simulink model "Simscape_Benchmark_SIM1"  (R2021a)
settings: Solver=ode45  StartTime=0.0  StopTime=PHASE.Ttotal  FixedStep=Benchmark.Sim.Tint  RelTol=1e-5  AbsTol=1e-6
undefined symbols (not defined in the file): Actuators, Analysis, antisym, Benchmark, Bus, Disturbance, FSM, IntialCond, ISOL, K_Coarse_disc_t, Kslew_opt_disc_zoh, Model, MPS, PAYLOAD, PHASE, PMA, RWIsol, RWS, SA, Sensors, Slew, slosh, thr, X, Y, Z
libraries: sm_lib x215, nesl_utility x148, simulink x65, cstblocks x36, sharedtransform x4, vrlib x3, RCTblocks x1
(part 4 of 9)

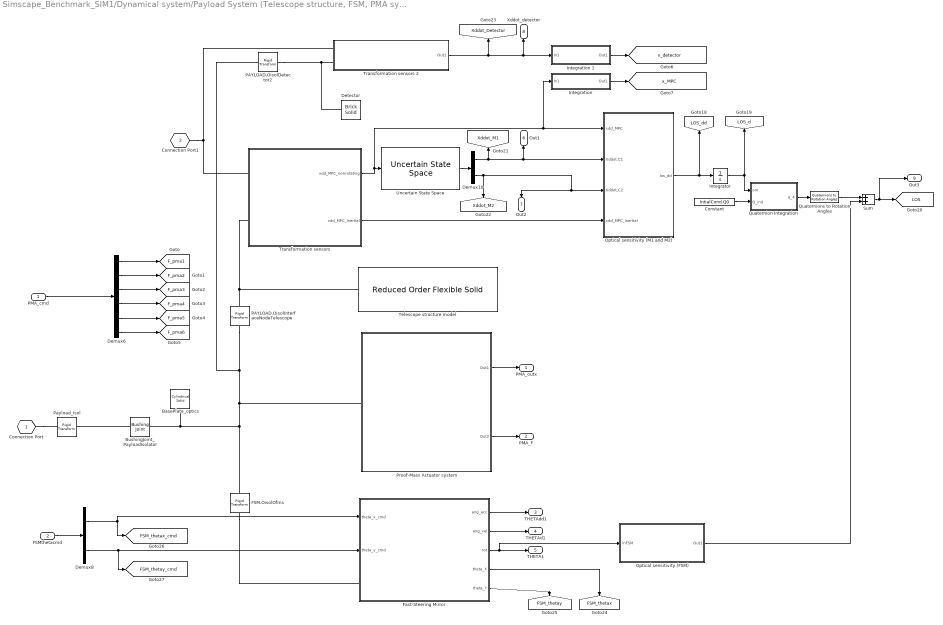
== system Simscape_Benchmark_SIM1/Dynamical system/Payload System (Telescope structure, FSM, PMA system, Isolator) ==
  PMA_cmd : Inport
  FSMthetacmd : Inport  Port=2
  BasePlate_optics : sm_lib/Body Elements/Cylindrical Solid  GraphicAmbientColor=[0.15 0.15 0.15 1.0]  BasedOnType=Density  CenterOfMass=[0;0;0]  CenterOfMassUnits=m  GraphicDiffuseColor=[0.0 0.2 0.6]  CylinderLength=ISOL.SIM.length  CylinderLengthUnits=m  CylinderRadius=ISOL.SIM.r_visualization  CylinderRadiusUnits=m  Density=1000  DensityUnits=kg/m^3  DoExposeReferenceFrame=off  GraphicEmissiveColor=[0.0 0.0 0.0 1.0]  ExportEntireGeometry=off  SerializedFrames=<Frames><Frame><Id>Frame1</Id><Value><Name>F1</Name><Origin><Source>GeometricFeature</Source><FeatureName>bottom surface</FeatureName></Origin><PrimaryAxis><DefinedDirection>+Z</DefinedDirection><Source>ReferenceFrame</Source><SourceDirection>+Z</SourceDirection><FeatureName></FeatureName></PrimaryAxis><SecondaryAxis><DefinedDirection>+X</DefinedDirection><Source>ReferenceFrame</Source><SourceDirection>+X</SourceDirection><FeatureName></FeatureName></SecondaryAxis></Value></Frame></Frames>  MarkerShape=Sphere  MarkerSize=10  GraphicType=FromGeometry  InertiaType=Custom  Mass=ISOL.m_simscape  MassUnits=kg  MomentsOfInertia=diag(ISOL.IatG_simscape)  MomentsOfInertiaUnits=kg*m^2  GraphicOpacity=0.4  ProductsOfInertia=[ISOL.IatG_simscape(2,3),ISOL.IatG_simscape(1,3),ISOL.IatG_simscape(1,2)]'  ProductsOfInertiaUnits=kg*m^2  GraphicShininess=75  GraphicSpecularColor=[0.5 0.5 0.5 1.0]  GraphicVisPropType=SimpleVisualProperties
  BushingJoint_PayloadIsolator : sm_lib/Joints/Bushing Joint  JointMode=Normal  SenseConstraintForce=off  SenseConstraintForceX=off  SenseConstraintForceY=off  SenseConstraintForceZ=off  SenseConstraintTorque=off  SenseConstraintTorqueX=off  SenseConstraintTorqueY=off  SenseConstraintTorqueZ=off  SenseTotalForce=off  SenseTotalForceX=off  SenseTotalForceY=off  SenseTotalForceZ=off  SenseTotalTorque=off  SenseTotalTorqueX=off  SenseTotalTorqueY=off  SenseTotalTorqueZ=off  CompositeWrenchDir=FollowerOnBase  CompositeWrenchFrame=BaseFrame  PxEquilibriumPosition=0  PxEquilibriumPositionUnits=m  PxSpringStiffness=ISOL.K(1,1)  PxSpringStiffnessUnits=N/m  PxDampingCoefficient=ISOL.D(1,1)  PxDampingCoefficientUnits=N/(m/s)  PxTorqueActuationMode=NoTorque  PxMotionActuationMode=ComputedMotion  PxSensePosition=off  PxSenseVelocity=off  PxSenseAcceleration=off  PxSenseTorqueForce=off  PxSenseLowerLimitTorqueForce=off  PxSenseUpperLimitTorqueForce=off  PxLowerLimitSpecify=off  PxLowerLimitBound=-1  PxLowerLimitBoundUnits=m  PxLowerLimitStiffness=1e6  PxLowerLimitStiffnessUnits=N/m  PxLowerLimitDamping=1e3  PxLowerLimitDampingUnits=N/(m/s)  PxLowerLimitTransitionRegionWidth=1e-4  PxLowerLimitTransitionRegionWidthUnits=m  PxUpperLimitSpecify=off  PxUpperLimitBound=1  PxUpperLimitBoundUnits=m  PxUpperLimitStiffness=1e6  PxUpperLimitStiffnessUnits=N/m  PxUpperLimitDamping=1e3  PxUpperLimitDampingUnits=N/(m/s)  PxUpperLimitTransitionRegionWidth=1e-4  PxUpperLimitTransitionRegionWidthUnits=m  PxPositionTargetSpecify=off  PxPositionTargetPriority=High  PxPositionTargetValue=0  PxPositionTargetValueUnits=m  PxVelocityTargetSpecify=off  PxVelocityTargetPriority=High  PxVelocityTargetValue=0  PxVelocityTargetValueUnits=m/s  PyEquilibriumPosition=0  PyEquilibriumPositionUnits=m  PySpringStiffness=ISOL.K(2,2)  PySpringStiffnessUnits=N/m  PyDampingCoefficient=ISOL.D(2,2)  PyDampingCoefficientUnits=N/(m/s)  PyTorqueActuationMode=NoTorque  PyMotionActuationMode=ComputedMotion  PySensePosition=off  PySenseVelocity=off  PySenseAcceleration=off  PySenseTorqueForce=off  PySenseLowerLimitTorqueForce=off  PySenseUpperLimitTorqueForce=off  PyLowerLimitSpecify=on  PyLowerLimitBound=-1  PyLowerLimitBoundUnits=m  PyLowerLimitStiffness=1e6  PyLowerLimitStiffnessUnits=N/m  PyLowerLimitDamping=1e3  PyLowerLimitDampingUnits=N/(m/s)  PyLowerLimitTransitionRegionWidth=1e-4  PyLowerLimitTransitionRegionWidthUnits=m  PyUpperLimitSpecify=off  PyUpperLimitBound=1  PyUpperLimitBoundUnits=m  PyUpperLimitStiffness=1e6  PyUpperLimitStiffnessUnits=N/m  PyUpperLimitDamping=1e3  PyUpperLimitDampingUnits=N/(m/s)  PyUpperLimitTransitionRegionWidth=1e-4  PyUpperLimitTransitionRegionWidthUnits=m  PyPositionTargetSpecify=off  PyPositionTargetPriority=High  PyPositionTargetValue=0  PyPositionTargetValueUnits=m  PyVelocityTargetSpecify=off  PyVelocityTargetPriority=High  PyVelocityTargetValue=0  PyVelocityTargetValueUnits=m/s  PzEquilibriumPosition=0  PzEquilibriumPositionUnits=m  PzSpringStiffness=ISOL.K(3,3)  PzSpringStiffnessUnits=N/m  PzDampingCoefficient=ISOL.D(3,3)  PzDampingCoefficientUnits=N/(m/s)  PzTorqueActuationMode=NoTorque  PzMotionActuationMode=ComputedMotion  PzSensePosition=off  PzSenseVelocity=off  PzSenseAcceleration=off  PzSenseTorqueForce=off  PzSenseLowerLimitTorqueForce=off  PzSenseUpperLimitTorqueForce=off  PzLowerLimitSpecify=off  PzLowerLimitBound=-1  PzLowerLimitBoundUnits=m  PzLowerLimitStiffness=1e6  PzLowerLimitStiffnessUnits=N/m  PzLowerLimitDamping=1e3  PzLowerLimitDampingUnits=N/(m/s)  PzLowerLimitTransitionRegionWidth=1e-4  PzLowerLimitTransitionRegionWidthUnits=m  PzUpperLimitSpecify=off  PzUpperLimitBound=1  PzUpperLimitBoundUnits=m  PzUpperLimitStiffness=1e6  PzUpperLimitStiffnessUnits=N/m  PzUpperLimitDamping=1e3  PzUpperLimitDampingUnits=N/(m/s)  PzUpperLimitTransitionRegionWidth=1e-4  PzUpperLimitTransitionRegionWidthUnits=m  PzPositionTargetSpecify=off  PzPositionTargetPriority=High  PzPositionTargetValue=0  PzPositionTargetValueUnits=m  PzVelocityTargetSpecify=off  PzVelocityTargetPriority=High  PzVelocityTargetValue=0  PzVelocityTargetValueUnits=m/s  RxEquilibriumPosition=0  RxEquilibriumPositionUnits=deg  RxSpringStiffness=ISOL.K(4,4)  RxSpringStiffnessUnits=N*m/rad  RxDampingCoefficient=ISOL.D(4,4)  RxDampingCoefficientUnits=N*m/(rad/s)  RxTorqueActuationMode=NoTorque  RxMotionActuationMode=ComputedMotion  RxSensePosition=off  RxSenseVelocity=off  RxSenseAcceleration=off  RxSenseTorqueForce=off  RxSenseLowerLimitTorqueForce=off  RxSenseUpperLimitTorqueForce=off  RxLowerLimitSpecify=off  RxLowerLimitBound=-90  RxLowerLimitBoundUnits=deg  RxLowerLimitStiffness=1e4  RxLowerLimitStiffnessUnits=N*m/deg  RxLowerLimitDamping=10  RxLowerLimitDampingUnits=N*m/(deg/s)  RxLowerLimitTransitionRegionWidth=0.1  RxLowerLimitTransitionRegionWidthUnits=deg  RxUpperLimitSpecify=off  RxUpperLimitBound=90  RxUpperLimitBoundUnits=deg  RxUpperLimitStiffness=1e4  RxUpperLimitStiffnessUnits=N*m/deg  RxUpperLimitDamping=10  RxUpperLimitDampingUnits=N*m/(deg/s)  RxUpperLimitTransitionRegionWidth=0.1  RxUpperLimitTransitionRegionWidthUnits=deg  RxPositionTargetSpecify=off  RxPositionTargetPriority=High  RxPositionTargetValue=0  RxPositionTargetValueUnits=deg  RxVelocityTargetSpecify=off  RxVelocityTargetPriority=High  RxVelocityTargetValue=0  RxVelocityTargetValueUnits=deg/s  RyEquilibriumPosition=0  RyEquilibriumPositionUnits=deg  RySpringStiffness=ISOL.K(5,5)  RySpringStiffnessUnits=N*m/rad  RyDampingCoefficient=ISOL.D(5,5)  RyDampingCoefficientUnits=N*m/(rad/s)  RyTorqueActuationMode=NoTorque  RyMotionActuationMode=ComputedMotion  RySensePosition=off  RySenseVelocity=off  RySenseAcceleration=off  RySenseTorqueForce=off  RySenseLowerLimitTorqueForce=off  RySenseUpperLimitTorqueForce=off  RyLowerLimitSpecify=off  RyLowerLimitBound=-90  RyLowerLimitBoundUnits=deg  RyLowerLimitStiffness=1e4  RyLowerLimitStiffnessUnits=N*m/deg  RyLowerLimitDamping=10  RyLowerLimitDampingUnits=N*m/(deg/s)  RyLowerLimitTransitionRegionWidth=0.1  RyLowerLimitTransitionRegionWidthUnits=deg  RyUpperLimitSpecify=off  RyUpperLimitBound=90  RyUpperLimitBoundUnits=deg  RyUpperLimitStiffness=1e4  RyUpperLimitStiffnessUnits=N*m/deg  RyUpperLimitDamping=10  RyUpperLimitDampingUnits=N*m/(deg/s)  RyUpperLimitTransitionRegionWidth=0.1  RyUpperLimitTransitionRegionWidthUnits=deg  RyPositionTargetSpecify=off  RyPositionTargetPriority=High  RyPositionTargetValue=0  RyPositionTargetValueUnits=deg  RyVelocityTargetSpecify=off  RyVelocityTargetPriority=High  RyVelocityTargetValue=0  RyVelocityTargetValueUnits=deg/s  RzEquilibriumPosition=0  RzEquilibriumPositionUnits=deg  RzSpringStiffness=ISOL.K(6,6)  RzSpringStiffnessUnits=N*m/rad  RzDampingCoefficient=ISOL.D(6,6)  RzDampingCoefficientUnits=N*m/(rad/s)  RzTorqueActuationMode=NoTorque  RzMotionActuationMode=ComputedMotion  RzSensePosition=off  RzSenseVelocity=off  RzSenseAcceleration=off  RzSenseTorqueForce=off  RzSenseLowerLimitTorqueForce=off  RzSenseUpperLimitTorqueForce=off  RzLowerLimitSpecify=off  RzLowerLimitBound=-90  RzLowerLimitBoundUnits=deg  RzLowerLimitStiffness=1e4  RzLowerLimitStiffnessUnits=N*m/deg  RzLowerLimitDamping=10  RzLowerLimitDampingUnits=N*m/(deg/s)  RzLowerLimitTransitionRegionWidth=0.1  RzLowerLimitTransitionRegionWidthUnits=deg  RzUpperLimitSpecify=off  RzUpperLimitBound=90  RzUpperLimitBoundUnits=deg  RzUpperLimitStiffness=1e4  RzUpperLimitStiffnessUnits=N*m/deg  RzUpperLimitDamping=10  RzUpperLimitDampingUnits=N*m/(deg/s)  RzUpperLimitTransitionRegionWidth=0.1  RzUpperLimitTransitionRegionWidthUnits=deg  RzPositionTargetSpecify=off  RzPositionTargetPriority=High  RzPositionTargetValue=0  RzPositionTargetValueUnits=deg  RzVelocityTargetSpecify=off  RzVelocityTargetPriority=High  RzVelocityTargetValue=0  RzVelocityTargetValueUnits=deg/s
  Constant : Constant  Value=IntialCond.Q0
  Demux10 : Demux  Outputs=[6,6]
  Demux6 : Demux  Outputs=6
  Demux8 : Demux  Outputs=2
  Detector : sm_lib/Body Elements/Brick Solid  GraphicAmbientColor=[0.15 0.15 0.15 1.0]  BasedOnType=Density  BrickDimensions=[0.05 0.05 0.002]  BrickDimensionUnits=m  CenterOfMass=[0 0 0]  CenterOfMassUnits=m  GraphicDiffuseColor=[1.0 1.0 0.0]  Density=0  DensityUnits=kg/m^3  DoExposeReferenceFrame=on  GraphicEmissiveColor=[0.0 0.0 0.0 1.0]  ExportEntireGeometry=off  SerializedFrames=<Frames/>  MarkerShape=Sphere  MarkerSize=10  GraphicType=FromGeometry  InertiaType=CalculateFromGeometry  Mass=1  MassUnits=kg  MomentsOfInertia=[1 1 1]  MomentsOfInertiaUnits=kg*m^2  GraphicOpacity=1.0  ProductsOfInertia=[0 0 0]  ProductsOfInertiaUnits=kg*m^2  GraphicShininess=75  GraphicSpecularColor=[0.5 0.5 0.5 1.0]  GraphicVisPropType=SimpleVisualProperties
  FSM.OisolOfms : sm_lib/Frames and Transforms/Rigid Transform  TranslationMethod=Cartesian  TranslationStandardOffset=0  TranslationLengthUnit=m  TranslationStandardAxis=+Z  TranslationCartesianOffset=FSM.OisolOfms  TranslationROffset=0  TranslationROffsetUnits=m  TranslationZOffset=0  TranslationZOffsetUnits=m  TranslationThetaOffset=0  TranslationThetaOffsetUnits=deg  RotationMethod=RotationMatrix  RotationAngleUnits=deg  RotationStandardAxis=+Z  RotationAngle=0.0  RotationArbitraryAxis=[0 0 1]  FollAlignAxisA=+X  BaseAlignAxisA=+Y  FollAlignAxisB=+Y  BaseAlignAxisB=+Z  RotationSequenceAxes=FollowerAxes  RotationSequence=XYX  RotationSequenceAngles=[0 0 0]  RotationSequenceAnglesUnits=deg  RotationMatrix=FSM.DCM
  Fast-Steering Mirror : Subsystem
  Integration : Subsystem
  Integration 1 : Subsystem
  Integrator : Integrator
  Optical sensitivity (FSM) : Subsystem
  Optical sensitivity (M1 and M2) : Subsystem
  PAYLOAD.OisolDetector2 : sm_lib/Frames and Transforms/Rigid Transform  TranslationMethod=Cartesian  TranslationStandardOffset=0  TranslationLengthUnit=m  TranslationStandardAxis=+Z  TranslationCartesianOffset=PAYLOAD.Detector.OisolDetector  TranslationROffset=0  TranslationROffsetUnits=m  TranslationZOffset=0  TranslationZOffsetUnits=m  TranslationThetaOffset=0  TranslationThetaOffsetUnits=deg  RotationMethod=RotationMatrix  RotationAngleUnits=deg  RotationStandardAxis=+Z  RotationAngle=0.0  RotationArbitraryAxis=[0 0 1]  FollAlignAxisA=+X  BaseAlignAxisA=+Y  FollAlignAxisB=+Y  BaseAlignAxisB=+Z  RotationSequenceAxes=FollowerAxes  RotationSequence=XYX  RotationSequenceAngles=[0 0 0]  RotationSequenceAnglesUnits=deg  RotationMatrix=PAYLOAD.Detector.DCM
  PAYLOAD.OisolInterfaceNodeTelescope : sm_lib/Frames and Transforms/Rigid Transform  TranslationMethod=Cartesian  TranslationStandardOffset=0  TranslationLengthUnit=m  TranslationStandardAxis=+Z  TranslationCartesianOffset=PAYLOAD.OisolInterfaceNodeTelescope  TranslationROffset=0  TranslationROffsetUnits=m  TranslationZOffset=0  TranslationZOffsetUnits=m  TranslationThetaOffset=0  TranslationThetaOffsetUnits=deg  RotationMethod=None  RotationAngleUnits=deg  RotationStandardAxis=+Z  RotationAngle=0.0  RotationArbitraryAxis=[0 0 1]  FollAlignAxisA=+X  BaseAlignAxisA=+Y  FollAlignAxisB=+Y  BaseAlignAxisB=+Z  RotationSequenceAxes=FollowerAxes  RotationSequence=XYX  RotationSequenceAngles=[0 0 0]  RotationSequenceAnglesUnits=deg  RotationMatrix=[1 0 0; 0 1 0; 0 0 1]
  Payload_Isol : sm_lib/Frames and Transforms/Rigid Transform  TranslationMethod=Cartesian  TranslationStandardOffset=0  TranslationLengthUnit=m  TranslationStandardAxis=+Z  TranslationCartesianOffset=ISOL.ObP  TranslationROffset=0  TranslationROffsetUnits=m  TranslationZOffset=0  TranslationZOffsetUnits=m  TranslationThetaOffset=0  TranslationThetaOffsetUnits=deg  RotationMethod=None  RotationAngleUnits=deg  RotationStandardAxis=+Z  RotationAngle=0.0  RotationArbitraryAxis=[0 0 1]  FollAlignAxisA=+X  BaseAlignAxisA=+Y  FollAlignAxisB=+Y  BaseAlignAxisB=+Z  RotationSequenceAxes=FollowerAxes  RotationSequence=XYX  RotationSequenceAngles=[0 0 0]  RotationSequenceAnglesUnits=deg  RotationMatrix=[1 0 0; 0 1 0; 0 0 1]
  Proof-Mass Actuator system : Subsystem
  Quaternion Integration : Subsystem
  Quaternions to Rotation Angles : sharedtransform/Quaternions to Rotation Angles  rotationOrder=XYZ  aMode=aMode
      settings: SourceProductBaseCode=AE,PW,DR,MT,UV,VE
  Sum : Sum
  Telescope structure model : sm_lib/Body Elements/Flexible Bodies/Reduced Order Flexible Solid  GraphicAmbientColor=[0.15 0.15 0.15 1.0]  GraphicDiffuseColor=[0.0 0.2 0.6]  DampingType=DampingMatrix  GraphicEmissiveColor=[0.0 0.0 0.0 1.0]  GeomFileName=file_telescope.stl  GraphicType=PartitionedGeometry  MassMatrix=PAYLOAD.Mrofs_telescopeSIMULATOR  NumberOfInterfaceFrames=1  GraphicOpacity=1  InterfaceFrameOrigins=PAYLOAD.coord_telescopeSIMULATOR  GraphicShininess=0  GraphicSpecularColor=[0.5 0.5 0.5 1.0]  StiffnessMatrix=PAYLOAD.Krofs_telescopeSIMULATOR  GeomUnitType=FromUnitSystem  VisRecursionLimit=3  GraphicVisPropType=SimpleVisualProperties  LengthUnit=m  MassUnit=kg  TimeUnit=s  UnitSystemType=SI  ProportionalDampingAlpha=0  ProportionalDampingBeta=0.001  UniformModalDampingRatio=0.005  DampingMatrix=PAYLOAD.Drofs_telescopeSIMULATOR
      settings: SourceProductBaseCode=MS
  Transformation sensors : Subsystem
  Transformation sensors 2 : Subsystem
  Uncertain State Space : RCTblocks/Uncertain State Space  Tag=USS  USystem=TF_telescope  UValue=PAYLOAD.Struct  X0=[]  uX0=[]
      settings: SourceProductBaseCode=RC
  Connection Port : PMIOPort  Tag=PMCPort  Side=Left
  Connection Port1 : PMIOPort  Tag=PMCPort  Port=2  Side=Left
  PMA_outx : Outport
  PMA_F : Outport  Port=2
  THETAdd1 : Outport  Port=3
  THETAd1 : Outport  Port=4
  THETA1 : Outport  Port=5
  Out1 : Outport  Port=6
  Out2 : Outport  Port=7
  Xddot_detector : Outport  Port=8
  Out3 : Outport  Port=9
  tag scope: FSM_thetax=global, FSM_thetax_cmd=global, FSM_thetay=global, FSM_thetay_cmd=global, F_pma1=global, F_pma2=global, F_pma3=global, F_pma4=global, F_pma5=global, F_pma6=global, LOS=global, LOS_d=global, LOS_dd=global, Xddot_Detector=global, Xddot_M1=global, Xddot_M2=global, x_MPC=global, x_detector=global
  wires:
  Demux6/2 -> [F_pma2]
  PMA_cmd/1 -> Demux6/1
  Demux6/1 -> [F_pma1]
  Demux6/6 -> [F_pma6]
  Demux6/5 -> [F_pma5]
  Demux6/3 -> [F_pma3]
  Demux6/4 -> [F_pma4]
  Demux8/2 -> [FSM_thetay_cmd], Fast-Steering Mirror/2(theta_y_cmd)
  Demux10/1 -> Optical sensitivity (M1 and M2)/2(Xddot,C1), Out1/1, [Xddot_M1]
  Optical sensitivity (M1 and M2)/1(los_dd) -> Integrator/1, [LOS_dd]
  Uncertain State Space/1 -> Demux10/1
  Demux8/1 -> [FSM_thetax_cmd], Fast-Steering Mirror/1(theta_x_cmd)
  Sum/1 -> Out3/1, [LOS]
  FSMthetacmd/1 -> Demux8/1
  Proof-Mass Actuator system/1(Out1) -> PMA_outx/1
  Proof-Mass Actuator system/2(Out2) -> PMA_F/1
  Fast-Steering Mirror/3(rot) -> Optical sensitivity (FSM)/1(inFSM), THETA1/1
  Fast-Steering Mirror/1(ang_acc) -> THETAdd1/1
  Fast-Steering Mirror/2(ang_vel) -> THETAd1/1
  Fast-Steering Mirror/4(theta_X) -> [FSM_thetax]
  Fast-Steering Mirror/5(theta_Y) -> [FSM_thetay]
  Demux10/2 -> Out2/1, Optical sensitivity (M1 and M2)/3(Xddot,C2), [Xddot_M2]
  Constant/1 -> Quaternion Integration/2(Q_init)
  Integrator/1 -> Quaternion Integration/1(om), [LOS_d]
  Quaternion Integration/1(q_4) -> Quaternions to Rotation Angles/1
  Optical sensitivity (FSM)/1(Out1) -> Sum/2
  Quaternions to Rotation Angles/1 -> Sum/1
  Integration/1(Out1) -> [x_MPC]
  Integration 1/1(Out1) -> [x_detector]
  Transformation sensors/1(xdd_MPC_nonrotating) -> Optical sensitivity (M1 and M2)/1(xdd_MPC), Integration/1(In1), Uncertain State Space/1
  Transformation sensors/2(xdd_MPC_Inertial) -> Optical sensitivity (M1 and M2)/4(xdd_MPC_Inertial)
  Transformation sensors 2/1(Out1) -> [Xddot_Detector], Xddot_detector/1, Integration 1/1(In1)
  connections:
  Connection Port/RConn1 -- Payload_Isol/LConn1
  FSM.OisolOfms/LConn1 -- PAYLOAD.OisolInterfaceNodeTelescope/LConn1 -- PAYLOAD.OisolDetector2/LConn1 -- Proof-Mass Actuator system/LConn1 -- BushingJoint_PayloadIsolator/RConn1 -- BasePlate_optics/LConn1
  BushingJoint_PayloadIsolator/LConn1 -- Payload_Isol/RConn1
  PAYLOAD.OisolInterfaceNodeTelescope/RConn1 -- Telescope structure model/LConn1 -- Transformation sensors/LConn2
  FSM.OisolOfms/RConn1 -- Fast-Steering Mirror/LConn1
  PAYLOAD.OisolDetector2/RConn1 -- Transformation sensors 2/LConn2 -- Detector/RConn1
  Connection Port1/RConn1 -- Transformation sensors/LConn1 -- Transformation sensors 2/LConn1

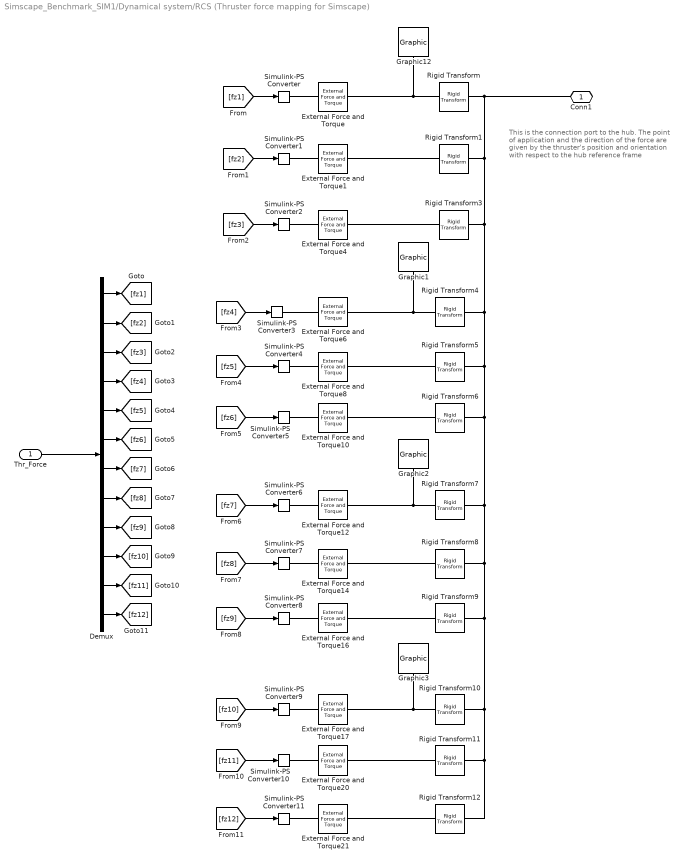
== system Simscape_Benchmark_SIM1/Dynamical system/RCS (Thruster force mapping for Simscape) ==
  note: This is the connection port to the hub. The point of application
      | and the direction of the force are given by the thruster's position
      | and orientation with respect to the hub reference frame
  Thr_Force : Inport
  Demux : Demux  Outputs=12
  External Force and Torque{,1,4,6,8,10,12,14,16..17,20..21} (12 alike) : sm_lib/Forces and Torques/External Force and Torque  ForceResolutionFrame=AttachedFrame  EnableForceX=off  EnableForceY=off  EnableForceZ=on  EnableForce=off  TorqueResolutionFrame=AttachedFrame  EnableTorqueX=off  EnableTorqueY=off  EnableTorqueZ=off  EnableTorque=off
  Graphic{1..3,12} (4 alike) : sm_lib/Body Elements/Graphic  GraphicType=Marker  MarkerShape=Frame  MarkerSize=15  GraphicVisPropType=SimpleVisualProperties  GraphicDiffuseColor=[0.0 0.0 0.8]  GraphicSpecularColor=[0.5 0.5 0.5 1.0]  GraphicAmbientColor=[0.15 0.15 0.15 1.0]  GraphicEmissiveColor=[0.0 0.0 0.0 1.0]  GraphicShininess=75  GraphicOpacity=1.0
  Rigid Transform : sm_lib/Frames and Transforms/Rigid Transform  TranslationMethod=Cartesian  TranslationStandardOffset=0  TranslationLengthUnit=m  TranslationStandardAxis=+Z  TranslationCartesianOffset=thr.sc_thrust_pos(:,1)  TranslationROffset=0  TranslationROffsetUnits=m  TranslationZOffset=0  TranslationZOffsetUnits=m  TranslationThetaOffset=0  TranslationThetaOffsetUnits=deg  RotationMethod=RotationMatrix  RotationAngleUnits=deg  RotationStandardAxis=+Z  RotationAngle=0.0  RotationArbitraryAxis=[0 0 1]  FollAlignAxisA=+X  BaseAlignAxisA=+Y  FollAlignAxisB=+Y  BaseAlignAxisB=+Z  RotationSequenceAxes=FollowerAxes  RotationSequence=XYX  RotationSequenceAngles=[0 0 0]  RotationSequenceAnglesUnits=deg  RotationMatrix=thr.FrameRot{1}
  Rigid Transform1 : sm_lib/Frames and Transforms/Rigid Transform  TranslationMethod=Cartesian  TranslationStandardOffset=0  TranslationLengthUnit=m  TranslationStandardAxis=+Z  TranslationCartesianOffset=thr.sc_thrust_pos(:,2)  TranslationROffset=0  TranslationROffsetUnits=m  TranslationZOffset=0  TranslationZOffsetUnits=m  TranslationThetaOffset=0  TranslationThetaOffsetUnits=deg  RotationMethod=RotationMatrix  RotationAngleUnits=deg  RotationStandardAxis=+Z  RotationAngle=0.0  RotationArbitraryAxis=[0 0 1]  FollAlignAxisA=+X  BaseAlignAxisA=+Y  FollAlignAxisB=+Y  BaseAlignAxisB=+Z  RotationSequenceAxes=FollowerAxes  RotationSequence=XYX  RotationSequenceAngles=[0 0 0]  RotationSequenceAnglesUnits=deg  RotationMatrix=thr.FrameRot{2}
  Rigid Transform10 : sm_lib/Frames and Transforms/Rigid Transform  TranslationMethod=Cartesian  TranslationStandardOffset=0  TranslationLengthUnit=m  TranslationStandardAxis=+Z  TranslationCartesianOffset=thr.sc_thrust_pos(:,10)  TranslationROffset=0  TranslationROffsetUnits=m  TranslationZOffset=0  TranslationZOffsetUnits=m  TranslationThetaOffset=0  TranslationThetaOffsetUnits=deg  RotationMethod=RotationMatrix  RotationAngleUnits=deg  RotationStandardAxis=+Z  RotationAngle=0.0  RotationArbitraryAxis=[0 0 1]  FollAlignAxisA=+X  BaseAlignAxisA=+Y  FollAlignAxisB=+Y  BaseAlignAxisB=+Z  RotationSequenceAxes=FollowerAxes  RotationSequence=XYX  RotationSequenceAngles=[0 0 0]  RotationSequenceAnglesUnits=deg  RotationMatrix=thr.FrameRot{10}
  Rigid Transform11 : sm_lib/Frames and Transforms/Rigid Transform  TranslationMethod=Cartesian  TranslationStandardOffset=0  TranslationLengthUnit=m  TranslationStandardAxis=+Z  TranslationCartesianOffset=thr.sc_thrust_pos(:,11)  TranslationROffset=0  TranslationROffsetUnits=m  TranslationZOffset=0  TranslationZOffsetUnits=m  TranslationThetaOffset=0  TranslationThetaOffsetUnits=deg  RotationMethod=RotationMatrix  RotationAngleUnits=deg  RotationStandardAxis=+Z  RotationAngle=0.0  RotationArbitraryAxis=[0 0 1]  FollAlignAxisA=+X  BaseAlignAxisA=+Y  FollAlignAxisB=+Y  BaseAlignAxisB=+Z  RotationSequenceAxes=FollowerAxes  RotationSequence=XYX  RotationSequenceAngles=[0 0 0]  RotationSequenceAnglesUnits=deg  RotationMatrix=thr.FrameRot{11}
  Rigid Transform12 : sm_lib/Frames and Transforms/Rigid Transform  TranslationMethod=Cartesian  TranslationStandardOffset=0  TranslationLengthUnit=m  TranslationStandardAxis=+Z  TranslationCartesianOffset=thr.sc_thrust_pos(:,12)  TranslationROffset=0  TranslationROffsetUnits=m  TranslationZOffset=0  TranslationZOffsetUnits=m  TranslationThetaOffset=0  TranslationThetaOffsetUnits=deg  RotationMethod=RotationMatrix  RotationAngleUnits=deg  RotationStandardAxis=+Z  RotationAngle=0.0  RotationArbitraryAxis=[0 0 1]  FollAlignAxisA=+X  BaseAlignAxisA=+Y  FollAlignAxisB=+Y  BaseAlignAxisB=+Z  RotationSequenceAxes=FollowerAxes  RotationSequence=XYX  RotationSequenceAngles=[0 0 0]  RotationSequenceAnglesUnits=deg  RotationMatrix=thr.FrameRot{12}
  Rigid Transform3 : sm_lib/Frames and Transforms/Rigid Transform  TranslationMethod=Cartesian  TranslationStandardOffset=0  TranslationLengthUnit=m  TranslationStandardAxis=+Z  TranslationCartesianOffset=thr.sc_thrust_pos(:,3)  TranslationROffset=0  TranslationROffsetUnits=m  TranslationZOffset=0  TranslationZOffsetUnits=m  TranslationThetaOffset=0  TranslationThetaOffsetUnits=deg  RotationMethod=RotationMatrix  RotationAngleUnits=deg  RotationStandardAxis=+Z  RotationAngle=0.0  RotationArbitraryAxis=[0 0 1]  FollAlignAxisA=+X  BaseAlignAxisA=+Y  FollAlignAxisB=+Y  BaseAlignAxisB=+Z  RotationSequenceAxes=FollowerAxes  RotationSequence=XYX  RotationSequenceAngles=[0 0 0]  RotationSequenceAnglesUnits=deg  RotationMatrix=thr.FrameRot{3}
  Rigid Transform4 : sm_lib/Frames and Transforms/Rigid Transform  TranslationMethod=Cartesian  TranslationStandardOffset=0  TranslationLengthUnit=m  TranslationStandardAxis=+Z  TranslationCartesianOffset=thr.sc_thrust_pos(:,4)  TranslationROffset=0  TranslationROffsetUnits=m  TranslationZOffset=0  TranslationZOffsetUnits=m  TranslationThetaOffset=0  TranslationThetaOffsetUnits=deg  RotationMethod=RotationMatrix  RotationAngleUnits=deg  RotationStandardAxis=+Z  RotationAngle=0.0  RotationArbitraryAxis=[0 0 1]  FollAlignAxisA=+X  BaseAlignAxisA=+Y  FollAlignAxisB=+Y  BaseAlignAxisB=+Z  RotationSequenceAxes=FollowerAxes  RotationSequence=XYX  RotationSequenceAngles=[0 0 0]  RotationSequenceAnglesUnits=deg  RotationMatrix=thr.FrameRot{4}
  Rigid Transform5 : sm_lib/Frames and Transforms/Rigid Transform  TranslationMethod=Cartesian  TranslationStandardOffset=0  TranslationLengthUnit=m  TranslationStandardAxis=+Z  TranslationCartesianOffset=thr.sc_thrust_pos(:,5)  TranslationROffset=0  TranslationROffsetUnits=m  TranslationZOffset=0  TranslationZOffsetUnits=m  TranslationThetaOffset=0  TranslationThetaOffsetUnits=deg  RotationMethod=RotationMatrix  RotationAngleUnits=deg  RotationStandardAxis=+Z  RotationAngle=0.0  RotationArbitraryAxis=[0 0 1]  FollAlignAxisA=+X  BaseAlignAxisA=+Y  FollAlignAxisB=+Y  BaseAlignAxisB=+Z  RotationSequenceAxes=FollowerAxes  RotationSequence=XYX  RotationSequenceAngles=[0 0 0]  RotationSequenceAnglesUnits=deg  RotationMatrix=thr.FrameRot{5}
  Rigid Transform6 : sm_lib/Frames and Transforms/Rigid Transform  TranslationMethod=Cartesian  TranslationStandardOffset=0  TranslationLengthUnit=m  TranslationStandardAxis=+Z  TranslationCartesianOffset=thr.sc_thrust_pos(:,6)  TranslationROffset=0  TranslationROffsetUnits=m  TranslationZOffset=0  TranslationZOffsetUnits=m  TranslationThetaOffset=0  TranslationThetaOffsetUnits=deg  RotationMethod=RotationMatrix  RotationAngleUnits=deg  RotationStandardAxis=+Z  RotationAngle=0.0  RotationArbitraryAxis=[0 0 1]  FollAlignAxisA=+X  BaseAlignAxisA=+Y  FollAlignAxisB=+Y  BaseAlignAxisB=+Z  RotationSequenceAxes=FollowerAxes  RotationSequence=XYX  RotationSequenceAngles=[0 0 0]  RotationSequenceAnglesUnits=deg  RotationMatrix=thr.FrameRot{6}
  Rigid Transform7 : sm_lib/Frames and Transforms/Rigid Transform  TranslationMethod=Cartesian  TranslationStandardOffset=0  TranslationLengthUnit=m  TranslationStandardAxis=+Z  TranslationCartesianOffset=thr.sc_thrust_pos(:,7)  TranslationROffset=0  TranslationROffsetUnits=m  TranslationZOffset=0  TranslationZOffsetUnits=m  TranslationThetaOffset=0  TranslationThetaOffsetUnits=deg  RotationMethod=RotationMatrix  RotationAngleUnits=deg  RotationStandardAxis=+Z  RotationAngle=0.0  RotationArbitraryAxis=[0 0 1]  FollAlignAxisA=+X  BaseAlignAxisA=+Y  FollAlignAxisB=+Y  BaseAlignAxisB=+Z  RotationSequenceAxes=FollowerAxes  RotationSequence=XYX  RotationSequenceAngles=[0 0 0]  RotationSequenceAnglesUnits=deg  RotationMatrix=thr.FrameRot{7}
  Rigid Transform8 : sm_lib/Frames and Transforms/Rigid Transform  TranslationMethod=Cartesian  TranslationStandardOffset=0  TranslationLengthUnit=m  TranslationStandardAxis=+Z  TranslationCartesianOffset=thr.sc_thrust_pos(:,8)  TranslationROffset=0  TranslationROffsetUnits=m  TranslationZOffset=0  TranslationZOffsetUnits=m  TranslationThetaOffset=0  TranslationThetaOffsetUnits=deg  RotationMethod=RotationMatrix  RotationAngleUnits=deg  RotationStandardAxis=+Z  RotationAngle=0.0  RotationArbitraryAxis=[0 0 1]  FollAlignAxisA=+X  BaseAlignAxisA=+Y  FollAlignAxisB=+Y  BaseAlignAxisB=+Z  RotationSequenceAxes=FollowerAxes  RotationSequence=XYX  RotationSequenceAngles=[0 0 0]  RotationSequenceAnglesUnits=deg  RotationMatrix=thr.FrameRot{8}
  Rigid Transform9 : sm_lib/Frames and Transforms/Rigid Transform  TranslationMethod=Cartesian  TranslationStandardOffset=0  TranslationLengthUnit=m  TranslationStandardAxis=+Z  TranslationCartesianOffset=thr.sc_thrust_pos(:,9)  TranslationROffset=0  TranslationROffsetUnits=m  TranslationZOffset=0  TranslationZOffsetUnits=m  TranslationThetaOffset=0  TranslationThetaOffsetUnits=deg  RotationMethod=RotationMatrix  RotationAngleUnits=deg  RotationStandardAxis=+Z  RotationAngle=0.0  RotationArbitraryAxis=[0 0 1]  FollAlignAxisA=+X  BaseAlignAxisA=+Y  FollAlignAxisB=+Y  BaseAlignAxisB=+Z  RotationSequenceAxes=FollowerAxes  RotationSequence=XYX  RotationSequenceAngles=[0 0 0]  RotationSequenceAnglesUnits=deg  RotationMatrix=thr.FrameRot{9}
  Simulink-PS Converter{,1..11} (12 alike) : nesl_utility/Simulink-PS Converter  PhysicalDomain=network_engine_domain  SubClassName=ps_input  LeftPortType=input  RightPortType=output  PseudoPeriodic=off  Frequencies=[]  NoiseDistribution=none  NoiseParameters=[]  Unit=1  AffineConversion=off  FilteringAndDerivatives=provide  SimscapeFilterOrder=1  InputFilterTimeConstant=0.001  UdotUserProvided=0
      settings: SourceProductBaseCode=PW,SS
  Conn1 : PMIOPort  Side=Right
  wires:
  Thr_Force/1 -> Demux/1
  Demux/1 -> [fz1]
  Demux/2 -> [fz2]
  Demux/3 -> [fz3]
  Demux/12 -> [fz12]
  Demux/11 -> [fz11]
  Demux/10 -> [fz10]
  Demux/9 -> [fz9]
  Demux/8 -> [fz8]
  Demux/7 -> [fz7]
  Demux/6 -> [fz6]
  Demux/5 -> [fz5]
  Demux/4 -> [fz4]
  [fz1] -> Simulink-PS Converter/1
  [fz2] -> Simulink-PS Converter1/1
  [fz3] -> Simulink-PS Converter2/1
  [fz4] -> Simulink-PS Converter3/1
  [fz5] -> Simulink-PS Converter4/1
  [fz6] -> Simulink-PS Converter5/1
  [fz7] -> Simulink-PS Converter6/1
  [fz8] -> Simulink-PS Converter7/1
  [fz9] -> Simulink-PS Converter8/1
  [fz10] -> Simulink-PS Converter9/1
  [fz11] -> Simulink-PS Converter10/1
  [fz12] -> Simulink-PS Converter11/1
  connections:
  Rigid Transform/RConn1 -- Graphic12/RConn1 -- External Force and Torque/RConn1
  Rigid Transform/LConn1 -- Rigid Transform9/LConn1 -- Rigid Transform12/LConn1 -- Rigid Transform11/LConn1 -- Rigid Transform10/LConn1 -- Rigid Transform8/LConn1 -- Rigid Transform7/LConn1 -- Rigid Transform6/LConn1 -- Rigid Transform5/LConn1 -- Rigid Transform4/LConn1 -- Rigid Transform3/LConn1 -- Rigid Transform1/LConn1 -- Conn1/RConn1
  Rigid Transform1/RConn1 -- External Force and Torque1/RConn1
  External Force and Torque4/RConn1 -- Rigid Transform3/RConn1
  Rigid Transform4/RConn1 -- Graphic1/RConn1 -- External Force and Torque6/RConn1
  Rigid Transform5/RConn1 -- External Force and Torque8/RConn1
  External Force and Torque10/RConn1 -- Rigid Transform6/RConn1
  Rigid Transform7/RConn1 -- Graphic2/RConn1 -- External Force and Torque12/RConn1
  External Force and Torque14/RConn1 -- Rigid Transform8/RConn1
  Rigid Transform10/RConn1 -- Graphic3/RConn1 -- External Force and Torque17/RConn1
  External Force and Torque16/RConn1 -- Rigid Transform9/RConn1
  External Force and Torque21/RConn1 -- Rigid Transform12/RConn1
  External Force and Torque20/RConn1 -- Rigid Transform11/RConn1
  Simulink-PS Converter/RConn1 -- External Force and Torque/LConn1
  Simulink-PS Converter1/RConn1 -- External Force and Torque1/LConn1
  Simulink-PS Converter2/RConn1 -- External Force and Torque4/LConn1
  Simulink-PS Converter3/RConn1 -- External Force and Torque6/LConn1
  Simulink-PS Converter4/RConn1 -- External Force and Torque8/LConn1
  External Force and Torque10/LConn1 -- Simulink-PS Converter5/RConn1
  External Force and Torque12/LConn1 -- Simulink-PS Converter6/RConn1
  Simulink-PS Converter7/RConn1 -- External Force and Torque14/LConn1
  Simulink-PS Converter8/RConn1 -- External Force and Torque16/LConn1
  Simulink-PS Converter9/RConn1 -- External Force and Torque17/LConn1
  External Force and Torque20/LConn1 -- Simulink-PS Converter10/RConn1
  External Force and Torque21/LConn1 -- Simulink-PS Converter11/RConn1

== system Simscape_Benchmark_SIM1/Dynamical system/RCS models ==
  Cmd_Torque : Inport
  Enable : EnablePort  StatesWhenEnabling=reset
  "Actuators.RCS.SelectFullModel " : Gain  Gain=Actuators.RCS.SelectFullModel
  Actuators.RCS.SelectIdeal : Gain  Gain=Actuators.RCS.SelectIdeal
  Actuators.RCS.SelectNoPWM : Gain  Gain=Actuators.RCS.SelectNoPWM
  Constant : Constant  Value=[0;0;0]
  Constant2 : Constant  Value=[0;0;0]
  Mux6 : Mux  Inputs=[3,3]
  RCS (thruster model) : Subsystem
  Sum1 : Sum
  F_thr : Outport  OutputWhenDisabled=reset  InitialOutput=zeros(thr.nb_thr,1)
  Wrench_ideal : Outport  Port=2  OutputWhenDisabled=reset  InitialOutput=zeros(6,1)
  n_thr_active : Outport  Port=3
  Thr_Force_NoPWM : Outport  Port=4
  wires:
  Actuators.RCS.SelectNoPWM/1 -> Sum1/2
  Sum1/1 -> F_thr/1
  Constant2/1 -> RCS (thruster model)/1(Cmd_force)
  Mux6/1 -> Actuators.RCS.SelectIdeal/1
  RCS (thruster model)/1(Thr_Force) -> "Actuators.RCS.SelectFullModel "/1
  "Actuators.RCS.SelectFullModel "/1 -> Sum1/1
  Cmd_Torque/1 -> Mux6/2, RCS (thruster model)/2(Cmd_Torque)
  Constant/1 -> Mux6/1
  RCS (thruster model)/2(Thr_Force_NoPWM) -> Thr_Force_NoPWM/1, Actuators.RCS.SelectNoPWM/1
  Actuators.RCS.SelectIdeal/1 -> Wrench_ideal/1
  RCS (thruster model)/3(Thr_activated) -> n_thr_active/1
